simulink model "VirtualDAQ"  (R2021b)
settings: Solver=VariableStepAuto  StartTime=0.0  StopTime=inf  MaxStep=0.001  RelTol=1e-3
PostLoadFcn:
  | % Resize the model window
  | set(0,"Units","pixels")
  | sSize = get(0,"screensize");
  | set_param(gcs,'location',...
  |     [1,sSize(4)*0.01,round(sSize(3)/2),sSize(4)*0.96]);
  | 
  | % Reset the zoom
  | set_param(gcs, 'ZoomFactor','FitSystem')
libraries: fl_lib x5, simulink x4, nesl_utility x3, ee_lib x1, dspxfrm3 x1
(part 2 of 2)

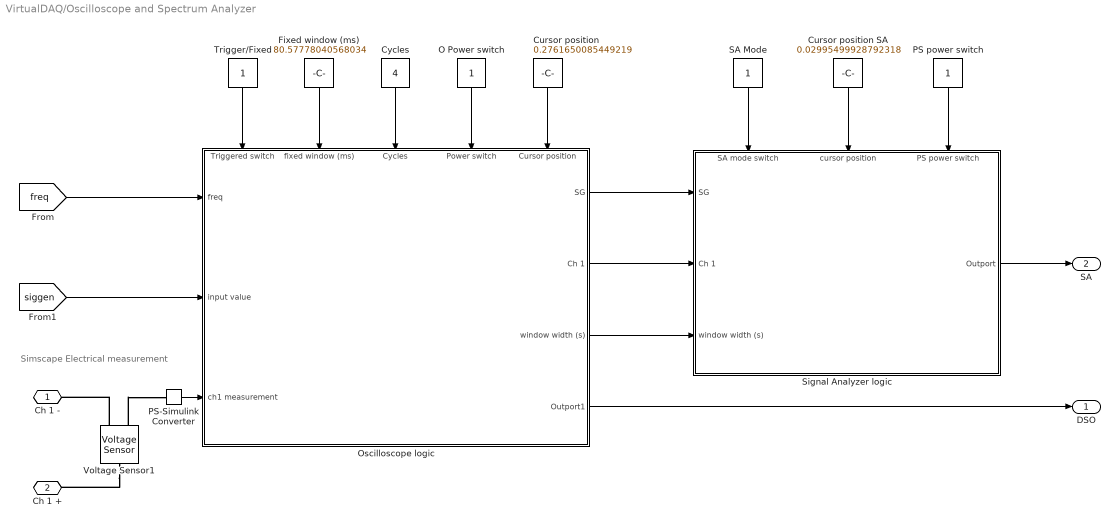
== system VirtualDAQ/Oscilloscope and Spectrum Analyzer ==
  note: Simscape Electrical
      | measurement
  Cursor position : Constant  Value=0.2761650085449219
  Cursor position SA : Constant  Value=0.02995499928792318
  Cycles : Constant  Value=4
  Fixed window (ms) : Constant  Value=80.57778040568034
  O Power switch : Constant
  Oscilloscope logic : Subsystem
      settings: PortSchema="{\"entries\":[{\"content\":{\"sides\":[{\"content\":{\"connectorIds\":[\"In1\",\"In2\",\"In3\"]},\"type\":\"ConnectorPlacement.EquallySpacedRectSide\",\"uuid\":\"f2d86859-c2b3-4aba-b253-ab7209c6bd09\"},{\"content\":{\"connectorIds\":[\"Out1\",\"Out2\",\"Out3\",\"Out4\"],\"side\":\"RIGHT\"},\"type\":\"ConnectorPlacement.EquallySpacedRectSide\",\"uuid\":\"576f7b6f-22d6-428c-bce1-54cbe46983a0\"},{\"content\":{\"connectorIds\":[\"In4\",\"In5\",\"In6\",\"In7\",\"In8\"],\"side\":\"TOP\"},\"type\":\"ConnectorPlacement.EquallySpacedRectSide\",\"uuid\":\"f25f0492-4e1a-4a19-8d4a-d023df9c7402\"}]},\"type\":\"ConnectorPlacement.EquallySpacedConnector\",\"uuid\":\"c0b076e3-46c8-476d-a521-4d4d737350f7\"}],\"packageUris\":[\"http://schema.mathworks.com/mf0/Connector/R2020b\"],\"version\":\"1.0\"}"
  PS power switch : Constant
  PS-Simulink Converter : nesl_utility/PS-Simulink Converter  PhysicalDomain=network_engine_domain  SubClassName=ps_output  LeftPortType=input  RightPortType=output  PseudoPeriodic=off  Frequencies=[]  Unit=inherit  AffineConversion=off
      settings: SourceProductBaseCode=PW,SS
  SA Mode : Constant
  Signal Analyzer logic : Subsystem
      settings: PortSchema="{\"entries\":[{\"content\":{\"sides\":[{\"content\":{\"connectorIds\":[\"In1\",\"In2\",\"In3\"]},\"type\":\"ConnectorPlacement.EquallySpacedRectSide\",\"uuid\":\"bb84044c-62d4-45e3-980b-d84da8bc32f8\"},{\"content\":{\"connectorIds\":[\"Out1\"],\"side\":\"RIGHT\"},\"type\":\"ConnectorPlacement.EquallySpacedRectSide\",\"uuid\":\"01e33b7c-25bd-4396-88e8-c83dc9c90d0e\"},{\"content\":{\"connectorIds\":[\"In4\",\"In5\",\"In6\"],\"side\":\"TOP\"},\"type\":\"ConnectorPlacement.EquallySpacedRectSide\",\"uuid\":\"0960ff1c-97c3-4c41-84a3-75686bdd4271\"}]},\"type\":\"ConnectorPlacement.EquallySpacedConnector\",\"uuid\":\"e23a09fd-d0ca-448f-9719-1e9fc283f1c0\"}],\"packageUris\":[\"http://schema.mathworks.com/mf0/Connector/R2020b\"],\"version\":\"1.0\"}"
  Trigger/Fixed : Constant
  Voltage Sensor1 : fl_lib/Electrical/Electrical Sensors/Voltage Sensor
  Ch 1 - : PMIOPort  Side=Left
  Ch 1 + : PMIOPort  Port=2  Side=Left
  DSO : Outport
  SA : Outport  Port=2
  wires:
  Trigger/Fixed/1 -> Oscilloscope logic/4(Triggered switch)
  Fixed window (ms)/1 -> Oscilloscope logic/5(fixed window (ms))
  Cycles/1 -> Oscilloscope logic/6(Cycles)
  O Power switch/1 -> Oscilloscope logic/7(Power switch)
  Cursor position/1 -> Oscilloscope logic/8(Cursor position)
  [freq] -> Oscilloscope logic/1(freq)
  [siggen] -> Oscilloscope logic/2(input value)
  Oscilloscope logic/4(Outport1) -> DSO/1
  SA Mode/1 -> Signal Analyzer logic/4(SA mode switch)
  Cursor position SA/1 -> Signal Analyzer logic/5(cursor position)
  PS power switch/1 -> Signal Analyzer logic/6(PS power switch)
  Oscilloscope logic/2(Ch 1) -> Signal Analyzer logic/2(Ch 1)
  Oscilloscope logic/1(SG) -> Signal Analyzer logic/1(SG)
  Oscilloscope logic/3(window width (s)) -> Signal Analyzer logic/3(window width (s))
  Signal Analyzer logic/1(Outport) -> SA/1
  PS-Simulink Converter/1 -> Oscilloscope logic/3(ch1 measurement)
  connections:
  Voltage Sensor1/RConn1 -- PS-Simulink Converter/LConn1
  Voltage Sensor1/LConn1 -- Ch 1 +/RConn1
  Voltage Sensor1/RConn2 -- Ch 1 -/RConn1

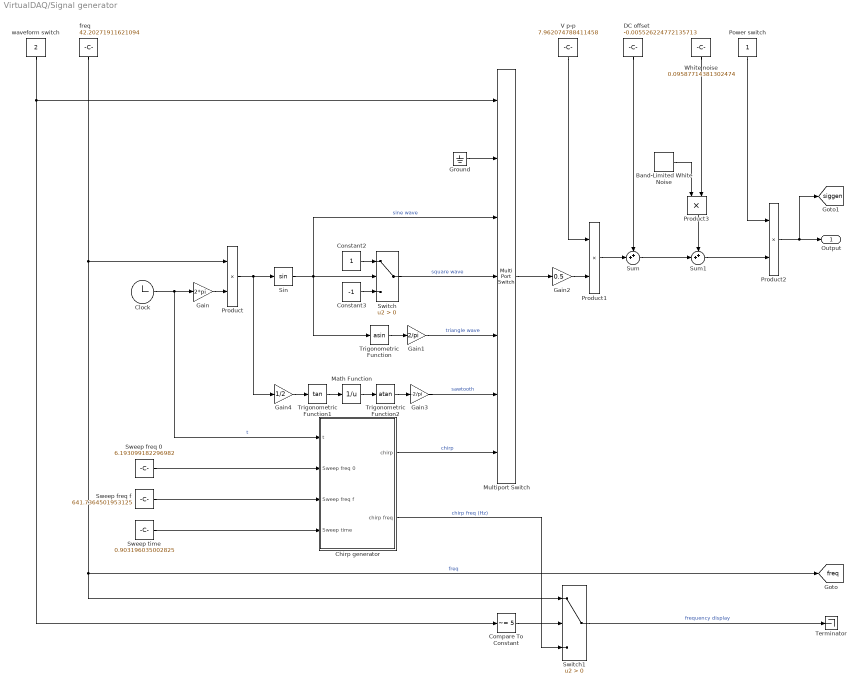
== system VirtualDAQ/Signal generator ==
  Band-Limited White Noise : simulink/Sources/Band-Limited White Noise  Cov=0.75e-6  Ts=0.5e-5  seed=[23341]
  Chirp generator : Subsystem
  Clock : Clock
  Compare To Constant : simulink/Logic and Bit Operations/Compare To Constant  relop=~=  const=5  OutDataTypeStr=boolean
  Constant2 : Constant  SampleTime=0
  Constant3 : Constant  Value=-1  SampleTime=0
  DC offset : Constant  Value=-0.005526224772135713
  Gain : Gain  Gain=2*pi
  Gain1 : Gain  Gain=2/pi
  Gain2 : Gain  Gain=0.5
  Gain3 : Gain  Gain=-2/pi
  Gain4 : Gain  Gain=1/2
  Ground : Ground
  Math Function : Math  Operator=reciprocal  SaturateOnIntegerOverflow=on
  Multiport Switch : MultiPortSwitch  DataPortOrder=Zero-based contiguous  Inputs=6  DiagnosticForDefault=None  zeroidx=on
  Power switch : Constant
  Product{,1..3} (4 alike) : Product
  Sin : Trigonometry
  Sum : Sum  Inputs=++|
  Sum1 : Sum  Inputs=++|
  Sweep freq 0 : Constant  Value=6.193099182296982
  Sweep freq f : Constant  Value=641.7364501953125
  Sweep time : Constant  Value=0.903196035002825
  Switch : Switch  Criteria=u2 > Threshold
  Switch1 : Switch  Criteria=u2 > Threshold
  Terminator : Terminator
  Trigonometric Function : Trigonometry  Operator=asin
  Trigonometric Function1 : Trigonometry  Operator=tan
  Trigonometric Function2 : Trigonometry  Operator=atan
  V p-p : Constant  Value=7.962074788411458  SampleTime=-1
  White noise : Constant  Value=0.09587714381302474
  freq : Constant  Value=42.20271911621094  SampleTime=0
  waveform switch : Constant  Value=2  SampleTime=0
  Output : Outport
  tag scope: freq=global, siggen=global
  wires:
  Sin/1 -> Multiport Switch/3, Trigonometric Function/1, Switch/2  "sine wave"
  freq/1 -> [freq], Switch1/1, Product/1  "freq"
  Clock/1 -> Chirp generator/1(t), Gain/1  "t"
  Ground/1 -> Multiport Switch/2
  Trigonometric Function/1 -> Gain1/1
  Constant2/1 -> Switch/1
  Constant3/1 -> Switch/3
  Gain2/1 -> Product1/2
  Product/1 -> Sin/1, Gain4/1
  Gain1/1 -> Multiport Switch/5  "triangle wave"
  Math Function/1 -> Trigonometric Function2/1
  Trigonometric Function1/1 -> Math Function/1
  Trigonometric Function2/1 -> Gain3/1
  Gain4/1 -> Trigonometric Function1/1
  Gain3/1 -> Multiport Switch/6  "sawtooth"
  V p-p/1 -> Product1/1
  Product1/1 -> Sum/2
  DC offset/1 -> Sum/1
  Switch/1 -> Multiport Switch/4  "square wave"
  Sum/1 -> Sum1/2
  Gain/1 -> Product/2
  Sweep time/1 -> Chirp generator/4(Sweep time)
  Chirp generator/1(chirp) -> Multiport Switch/7  "chirp"
  Sweep freq 0/1 -> Chirp generator/2(Sweep freq 0)
  Sweep freq f/1 -> Chirp generator/3(Sweep freq f)
  Compare To Constant/1 -> Switch1/2
  waveform switch/1 -> Compare To Constant/1, Multiport Switch/1
  Chirp generator/2(chirp freq) -> Switch1/3  "chirp freq (Hz)"
  Switch1/1 -> Terminator/1  "frequency display"
  Band-Limited White Noise/1 -> Product3/1
  White noise/1 -> Product3/2
  Product3/1 -> Sum1/1
  Power switch/1 -> Product2/1
  Sum1/1 -> Product2/2
  Product2/1 -> [siggen], Output/1
  Multiport Switch/1 -> Gain2/1

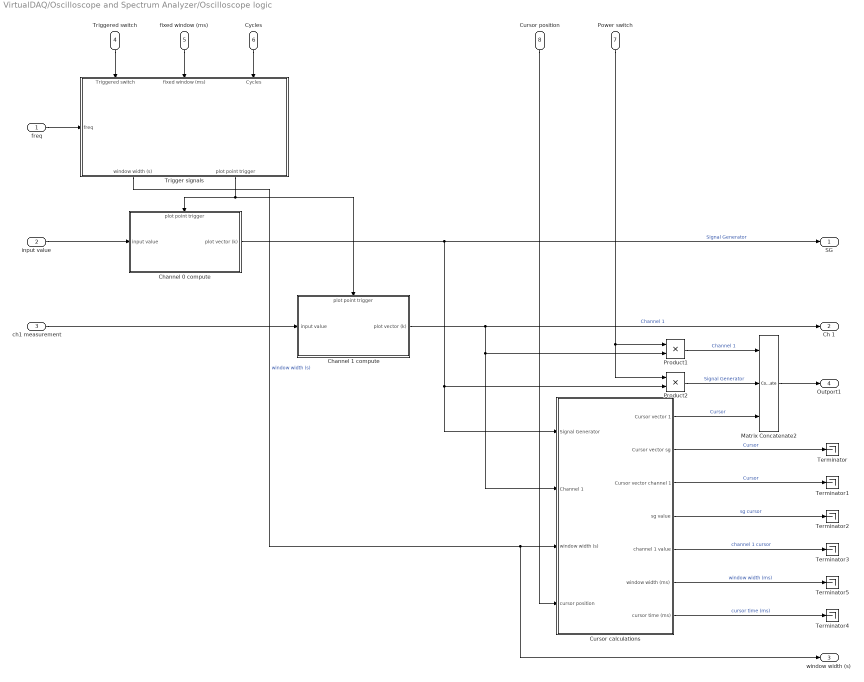
== system VirtualDAQ/Oscilloscope and Spectrum Analyzer/Oscilloscope logic ==
  freq : Inport
  input value : Inport  Port=2
  ch1 measurement : Inport  Port=3
  Triggered switch : Inport  Port=4
  fixed window (ms) : Inport  Port=5
  Cycles : Inport  Port=6
  Power switch : Inport  Port=7
  Cursor position : Inport  Port=8
  Channel 0 compute : Subsystem
      settings: PortSchema="{\"entries\":[{\"content\":{\"sides\":[{\"content\":{\"connectorIds\":[\"In1\"]},\"type\":\"ConnectorPlacement.EquallySpacedRectSide\",\"uuid\":\"56eea059-d5e9-4d95-b7d9-83a317b3103e\"},{\"content\":{\"connectorIds\":[\"Out1\"],\"side\":\"RIGHT\"},\"type\":\"ConnectorPlacement.EquallySpacedRectSide\",\"uuid\":\"fd8b8cd5-6def-4d8f-87ca-646372cc7fbe\"},{\"content\":{\"connectorIds\":[\"In2\"],\"side\":\"TOP\"},\"type\":\"ConnectorPlacement.EquallySpacedRectSide\",\"uuid\":\"3d9c38ee-b24b-466c-a7ac-a6d8a7456d51\"},{\"content\":{\"connectorIds\":[],\"side\":\"BOTTOM\"},\"type\":\"ConnectorPlacement.EquallySpacedRectSide\",\"uuid\":\"336136fa-2514-49ab-9e17-88caaca7366c\"}]},\"type\":\"ConnectorPlacement.EquallySpacedConnector\",\"uuid\":\"1d9824a8-6efd-49ff-b082-cf2ede19b4fd\"}],\"packageUris\":[\"http://schema.mathworks.com/mf0/Connector/R2020b\"],\"version\":\"1.0\"}"
  Channel 1 compute : Subsystem
      settings: PortSchema="{\"entries\":[{\"content\":{\"sides\":[{\"content\":{\"connectorIds\":[\"In1\"]},\"type\":\"ConnectorPlacement.EquallySpacedRectSide\",\"uuid\":\"56eea059-d5e9-4d95-b7d9-83a317b3103e\"},{\"content\":{\"connectorIds\":[\"Out1\"],\"side\":\"RIGHT\"},\"type\":\"ConnectorPlacement.EquallySpacedRectSide\",\"uuid\":\"fd8b8cd5-6def-4d8f-87ca-646372cc7fbe\"},{\"content\":{\"connectorIds\":[\"In2\"],\"side\":\"TOP\"},\"type\":\"ConnectorPlacement.EquallySpacedRectSide\",\"uuid\":\"3d9c38ee-b24b-466c-a7ac-a6d8a7456d51\"},{\"content\":{\"connectorIds\":[],\"side\":\"BOTTOM\"},\"type\":\"ConnectorPlacement.EquallySpacedRectSide\",\"uuid\":\"336136fa-2514-49ab-9e17-88caaca7366c\"}]},\"type\":\"ConnectorPlacement.EquallySpacedConnector\",\"uuid\":\"1d9824a8-6efd-49ff-b082-cf2ede19b4fd\"}],\"packageUris\":[\"http://schema.mathworks.com/mf0/Connector/R2020b\"],\"version\":\"1.0\"}"
  Cursor calculations : Subsystem
  Matrix Concatenate2 : Concatenate  NumInputs=3  Mode=Multidimensional array  ConcatenateDimension=2
  Product1 : Product
  Product2 : Product
  Terminator{,1..5} (6 alike) : Terminator
  Trigger signals : Subsystem
      settings: PortSchema="{\"entries\":[{\"content\":{\"sides\":[{\"content\":{\"connectorIds\":[\"In1\"]},\"type\":\"ConnectorPlacement.EquallySpacedRectSide\",\"uuid\":\"b92255b7-066e-487b-9e0c-e19692fc940f\"},{\"content\":{\"connectorIds\":[],\"side\":\"RIGHT\"},\"type\":\"ConnectorPlacement.EquallySpacedRectSide\",\"uuid\":\"cb964d42-f40b-466c-b45b-853437324272\"},{\"content\":{\"connectorIds\":[\"In2\",\"In3\",\"In4\"],\"side\":\"TOP\"},\"type\":\"ConnectorPlacement.EquallySpacedRectSide\",\"uuid\":\"e1027385-b295-47a3-ae7d-2e3bb07fa1de\"},{\"content\":{\"connectorIds\":[\"Out1\",\"Out2\"],\"side\":\"BOTTOM\"},\"type\":\"ConnectorPlacement.EquallySpacedRectSide\",\"uuid\":\"c27dc584-c0ba-4e72-b8bf-7374d1985911\"}]},\"type\":\"ConnectorPlacement.EquallySpacedConnector\",\"uuid\":\"1db11e79-2cf0-4841-86d9-651820ebc8ee\"}],\"packageUris\":[\"http://schema.mathworks.com/mf0/Connector/R2020b\"],\"version\":\"1.0\"}"
  SG : Outport
  Ch 1 : Outport  Port=2
  window width (s) : Outport  Port=3
  Outport1 : Outport  Port=4
  wires:
  Channel 0 compute/1(plot vector (k)) -> Cursor calculations/1(Signal Generator), Product2/2, SG/1  "Signal Generator"
  Power switch/1 -> Product2/1, Product1/1
  Trigger signals/2(plot point trigger) -> Channel 0 compute/2(plot point trigger), Channel 1 compute/2(plot point trigger)
  Trigger signals/1(window width (s)) -> window width (s)/1, Cursor calculations/3(window width (s))  "window width (s)"
  Channel 1 compute/1(plot vector (k)) -> Cursor calculations/2(Channel 1), Product1/2, Ch 1/1  "Channel 1"
  Cursor calculations/2(Cursor vector sg) -> Terminator/1  "Cursor"
  Cursor calculations/7(cursor time (ms)) -> Terminator4/1  "cursor time (ms)"
  Cursor calculations/4(sg value) -> Terminator2/1  "sg cursor"
  Cursor calculations/3(Cursor vector channel 1) -> Terminator1/1  "Cursor"
  Cursor calculations/5(channel 1 value) -> Terminator3/1  "channel 1 cursor"
  fixed window (ms)/1 -> Trigger signals/3(fixed window (ms))
  Cursor calculations/1(Cursor vector 1) -> Matrix Concatenate2/3  "Cursor"
  Product1/1 -> Matrix Concatenate2/1  "Channel 1"
  Cursor calculations/6(window width (ms)) -> Terminator5/1  "window width (ms)"
  Product2/1 -> Matrix Concatenate2/2  "Signal Generator"
  Triggered switch/1 -> Trigger signals/2(Triggered switch)
  input value/1 -> Channel 0 compute/1(input value)
  Cycles/1 -> Trigger signals/4(Cycles)
  freq/1 -> Trigger signals/1(freq)
  Matrix Concatenate2/1 -> Outport1/1
  Cursor position/1 -> Cursor calculations/4(cursor position)
  ch1 measurement/1 -> Channel 1 compute/1(input value)

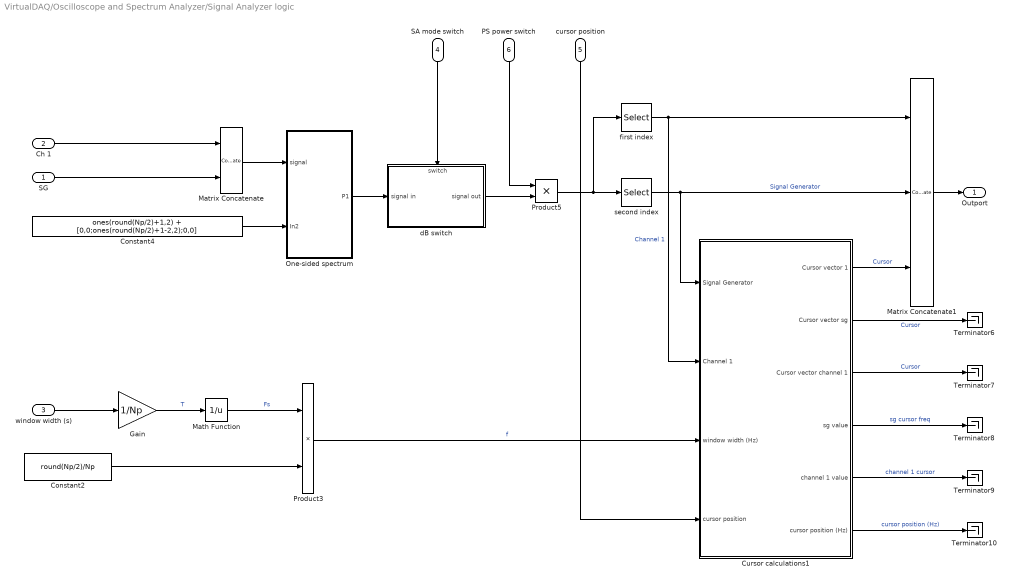
== system VirtualDAQ/Oscilloscope and Spectrum Analyzer/Signal Analyzer logic ==
  SG : Inport
  Ch 1 : Inport  Port=2
  window width (s) : Inport  Port=3
  SA mode switch : Inport  Port=4
  cursor position : Inport  Port=5
  PS power switch : Inport  Port=6
  Constant2 : Constant  Value=round(Np/2)/Np
  Constant4 : Constant  Value=ones(round(Np/2)+1,2) + [0,0;ones(round(Np/2)+1-2,2);0,0]
  Cursor calculations1 : Subsystem
  Gain : Gain  Gain=1/Np
  Math Function : Math  Operator=reciprocal  SaturateOnIntegerOverflow=on
  Matrix Concatenate : Concatenate  Mode=Multidimensional array  ConcatenateDimension=2
  Matrix Concatenate1 : Concatenate  NumInputs=3  Mode=Multidimensional array  ConcatenateDimension=2
  One-sided spectrum : Subsystem
  Product3 : Product
  Product5 : Product
  Terminator{6..10} (5 alike) : Terminator
  dB switch : Subsystem
      settings: PortSchema="{\"entries\":[{\"content\":{\"sides\":[{\"content\":{\"connectorIds\":[\"In1\"]},\"type\":\"ConnectorPlacement.EquallySpacedRectSide\",\"uuid\":\"731d6ea0-13ec-4437-83d3-031943873cb5\"},{\"content\":{\"connectorIds\":[\"Out1\"],\"side\":\"RIGHT\"},\"type\":\"ConnectorPlacement.EquallySpacedRectSide\",\"uuid\":\"4a6928d1-e59a-43a6-b645-c5c732165a4d\"},{\"content\":{\"connectorIds\":[\"In2\"],\"side\":\"TOP\"},\"type\":\"ConnectorPlacement.EquallySpacedRectSide\",\"uuid\":\"01c58549-3c91-47fa-983a-e1347000b7e8\"}]},\"type\":\"ConnectorPlacement.EquallySpacedConnector\",\"uuid\":\"72ae96ee-473e-47d4-a3f7-467fafe8904d\"}],\"packageUris\":[\"http://schema.mathworks.com/mf0/Connector/R2020b\"],\"version\":\"1.0\"}"
  first index : Selector  NumberOfDimensions=2  InputPortWidth=3  IndexOptions=Select all,Index vector (dialog)  Indices=[1 3],1  OutputSizes=1,1
  second index : Selector  NumberOfDimensions=2  InputPortWidth=3  IndexOptions=Select all,Index vector (dialog)  Indices=[1 3],2  OutputSizes=1,1
  Outport : Outport
  wires:
  Constant2/1 -> Product3/2
  Math Function/1 -> Product3/1  "Fs"
  Gain/1 -> Math Function/1  "T"
  Product3/1 -> Cursor calculations1/3(window width (Hz))  "f"
  Cursor calculations1/6(cursor position (Hz)) -> Terminator10/1  "cursor position (Hz)"
  Matrix Concatenate/1 -> One-sided spectrum/1(signal)
  first index/1 -> Cursor calculations1/2(Channel 1), Matrix Concatenate1/1  "Channel 1"
  Cursor calculations1/5(channel 1 value) -> Terminator9/1  "channel 1 cursor"
  Cursor calculations1/1(Cursor vector 1) -> Matrix Concatenate1/3  "Cursor"
  second index/1 -> Matrix Concatenate1/2, Cursor calculations1/1(Signal Generator)  "Signal Generator"
  Constant4/1 -> One-sided spectrum/2(In2)
  Cursor calculations1/3(Cursor vector channel 1) -> Terminator7/1  "Cursor"
  window width (s)/1 -> Gain/1
  Product5/1 -> first index/1, second index/1
  PS power switch/1 -> Product5/1
  One-sided spectrum/1(P1) -> dB switch/1(signal in)
  Cursor calculations1/4(sg value) -> Terminator8/1  "sg cursor freq"
  Cursor calculations1/2(Cursor vector sg) -> Terminator6/1  "Cursor"
  SG/1 -> Matrix Concatenate/2
  dB switch/1(signal out) -> Product5/2
  Ch 1/1 -> Matrix Concatenate/1
  cursor position/1 -> Cursor calculations1/4(cursor position)
  SA mode switch/1 -> dB switch/2(switch)
  Matrix Concatenate1/1 -> Outport/1

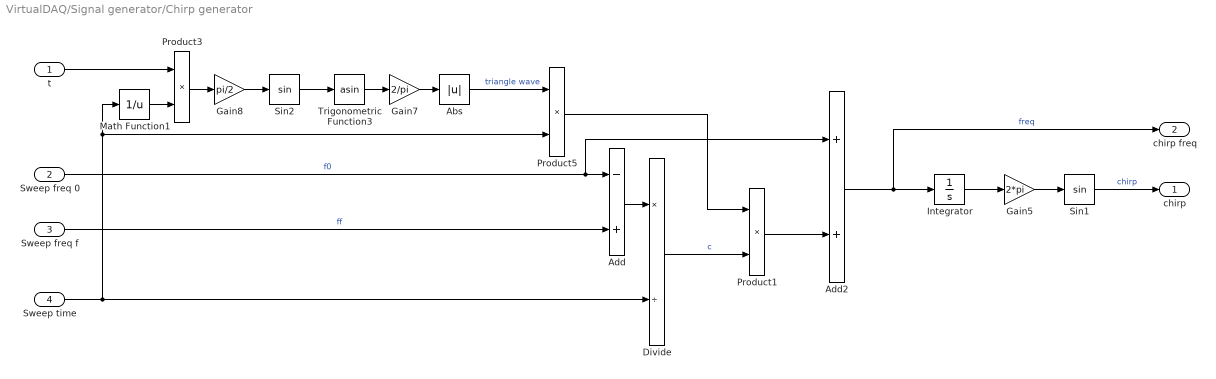
== system VirtualDAQ/Signal generator/Chirp generator ==
  t : Inport
  Sweep freq 0 : Inport  Port=2
  Sweep freq f : Inport  Port=3
  Sweep time : Inport  Port=4
  Abs : Abs
  Add : Sum  Inputs=-+
  Add2 : Sum
  Divide : Product  Inputs=*/
  Gain5 : Gain  Gain=2*pi
  Gain7 : Gain  Gain=2/pi
  Gain8 : Gain  Gain=pi/2
  Integrator : Integrator
  Math Function1 : Math  Operator=reciprocal  SaturateOnIntegerOverflow=on
  Product1 : Product
  Product3 : Product
  Product5 : Product
  Sin1 : Trigonometry
  Sin2 : Trigonometry
  Trigonometric Function3 : Trigonometry  Operator=asin
  chirp : Outport
  chirp freq : Outport  Port=2
  wires:
  Add/1 -> Divide/1
  Gain5/1 -> Sin1/1
  Gain8/1 -> Sin2/1
  Divide/1 -> Product1/2  "c"
  Sweep time/1 -> Divide/2, Product5/2, Math Function1/1
  Gain7/1 -> Abs/1
  t/1 -> Product3/1
  Sin2/1 -> Trigonometric Function3/1
  Trigonometric Function3/1 -> Gain7/1
  Math Function1/1 -> Product3/2
  Sin1/1 -> chirp/1  "chirp"
  Sweep freq 0/1 -> Add2/1, Add/1  "f0"
  Sweep freq f/1 -> Add/2  "ff"
  Product1/1 -> Add2/2
  Integrator/1 -> Gain5/1
  Add2/1 -> chirp freq/1, Integrator/1  "freq"
  Product3/1 -> Gain8/1
  Abs/1 -> Product5/1  "triangle wave"
  Product5/1 -> Product1/1

== system VirtualDAQ/Oscilloscope and Spectrum Analyzer/Oscilloscope logic/Channel 0 compute ==
  note: This level stores the plot values inside the delay block
  input value : Inport
  plot point trigger : Inport  Port=2
  Rate Transition2 : RateTransition  InitialCondition=zeros(Np,1)  OutPortSampleTime=1/refreshRate
  Triggered Subsystem : Subsystem  TreatAsAtomicUnit=on
  plot vector values : UnitDelay  InitialCondition=zeros(Np,1)  SampleTime=-1  HasFrameUpgradeWarning=on
  plot vector (k) : Outport
  wires:
  plot point trigger/1 -> Triggered Subsystem/Trigger
  Triggered Subsystem/1(plot vector (k)) -> Rate Transition2/1, plot vector values/1
  input value/1 -> Triggered Subsystem/1(input value)
  Rate Transition2/1 -> plot vector (k)/1
  plot vector values/1 -> Triggered Subsystem/2(plot vector (k-1))

== system VirtualDAQ/Oscilloscope and Spectrum Analyzer/Oscilloscope logic/Channel 1 compute ==
  note: This level stores the plot values inside the delay block
  input value : Inport
  plot point trigger : Inport  Port=2
  Rate Transition2 : RateTransition  InitialCondition=zeros(Np,1)  OutPortSampleTime=1/refreshRate
  Triggered Subsystem : Subsystem  TreatAsAtomicUnit=on
  plot vector values : UnitDelay  InitialCondition=zeros(Np,1)  SampleTime=-1  HasFrameUpgradeWarning=on
  plot vector (k) : Outport
  wires:
  plot point trigger/1 -> Triggered Subsystem/Trigger
  Triggered Subsystem/1(plot vector (k)) -> Rate Transition2/1, plot vector values/1
  input value/1 -> Triggered Subsystem/1(input value)
  Rate Transition2/1 -> plot vector (k)/1
  plot vector values/1 -> Triggered Subsystem/2(plot vector (k-1))

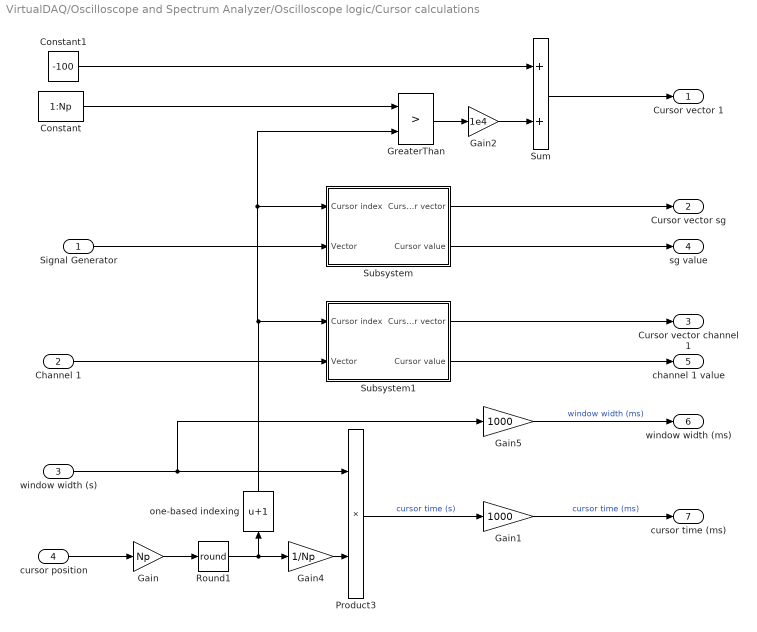
== system VirtualDAQ/Oscilloscope and Spectrum Analyzer/Oscilloscope logic/Cursor calculations ==
  Signal Generator : Inport
  Channel 1 : Inport  Port=2
  window width (s) : Inport  Port=3
  cursor position : Inport  Port=4
  Constant : Constant  Value=1:Np
  Constant1 : Constant  Value=-100
  Gain : Gain  Gain=Np
  Gain1 : Gain  Gain=1000
  Gain2 : Gain  Gain=1e4
  Gain4 : Gain  Gain=1/Np
  Gain5 : Gain  Gain=1000
  GreaterThan : RelationalOperator  Operator=>  OutDataTypeStr=boolean  RndMeth=Simplest
  Product3 : Product
  Round1 : Rounding  Operator=round
  Subsystem : Subsystem
  Subsystem1 : Subsystem
  Sum : Sum
  one-based indexing : Bias  Bias=1
  Cursor vector 1 : Outport
  Cursor vector sg : Outport  Port=2
  Cursor vector channel 1 : Outport  Port=3
  sg value : Outport  Port=4
  channel 1 value : Outport  Port=5
  window width (ms) : Outport  Port=6
  cursor time (ms) : Outport  Port=7
  wires:
  cursor position/1 -> Gain/1
  Constant/1 -> GreaterThan/1
  Product3/1 -> Gain1/1  "cursor time (s)"
  Gain1/1 -> cursor time (ms)/1  "cursor time (ms)"
  GreaterThan/1 -> Gain2/1
  Sum/1 -> Cursor vector 1/1
  Gain2/1 -> Sum/2
  Subsystem1/2(Cursor value) -> channel 1 value/1
  Constant1/1 -> Sum/1
  Gain/1 -> Round1/1
  Gain4/1 -> Product3/2
  Channel 1/1 -> Subsystem1/2(Vector)
  Subsystem1/1("Cursor vector ") -> Cursor vector channel 1/1
  Round1/1 -> Gain4/1, one-based indexing/1
  window width (s)/1 -> Gain5/1, Product3/1
  Gain5/1 -> window width (ms)/1  "window width (ms)"
  Signal Generator/1 -> Subsystem/2(Vector)
  Subsystem/1("Cursor vector ") -> Cursor vector sg/1
  Subsystem/2(Cursor value) -> sg value/1
  one-based indexing/1 -> GreaterThan/2, Subsystem/1(Cursor index), Subsystem1/1(Cursor index)

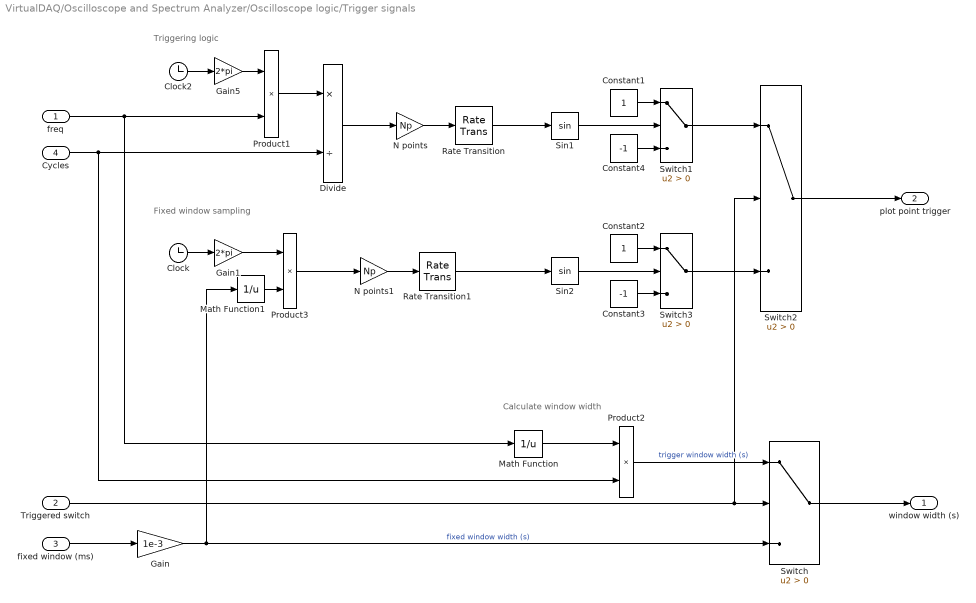
== system VirtualDAQ/Oscilloscope and Spectrum Analyzer/Oscilloscope logic/Trigger signals ==
  note: Calculate window width
  note: Triggering logic
  note: Fixed window sampling
  freq : Inport
  Triggered switch : Inport  Port=2
  fixed window (ms) : Inport  Port=3
  Cycles : Inport  Port=4
  Clock : Clock
  Clock2 : Clock
  Constant1 : Constant  SampleTime=0
  Constant2 : Constant  SampleTime=0
  Constant3 : Constant  Value=-1  SampleTime=0
  Constant4 : Constant  Value=-1  SampleTime=0
  Divide : Product  Inputs=*/
  Gain : Gain  Gain=1e-3
  Gain1 : Gain  Gain=2*pi
  Gain5 : Gain  Gain=2*pi
  Math Function : Math  Operator=reciprocal  SaturateOnIntegerOverflow=on
  Math Function1 : Math  Operator=reciprocal  SaturateOnIntegerOverflow=on
  N points : Gain  Gain=Np
  N points1 : Gain  Gain=Np
  Product1 : Product
  Product2 : Product
  Product3 : Product
  Rate Transition : RateTransition  OutPortSampleTime=plot_dt
  Rate Transition1 : RateTransition  OutPortSampleTime=plot_dt
  Sin1 : Trigonometry
  Sin2 : Trigonometry
  Switch{,1..3} (4 alike) : Switch  Criteria=u2 > Threshold
  window width (s) : Outport
  plot point trigger : Outport  Port=2
  wires:
  Gain5/1 -> Product1/1
  Constant4/1 -> Switch1/3
  Clock2/1 -> Gain5/1
  Sin1/1 -> Switch1/2
  Constant1/1 -> Switch1/1
  Product1/1 -> Divide/1
  Divide/1 -> N points/1
  N points/1 -> Rate Transition/1
  Rate Transition/1 -> Sin1/1
  Switch2/1 -> plot point trigger/1
  Triggered switch/1 -> Switch/2, Switch2/2
  Product2/1 -> Switch/1  "trigger window width (s)"
  freq/1 -> Product1/2, Math Function/1
  Cycles/1 -> Divide/2, Product2/2
  Math Function/1 -> Product2/1
  fixed window (ms)/1 -> Gain/1
  Switch/1 -> window width (s)/1
  Switch1/1 -> Switch2/1
  N points1/1 -> Rate Transition1/1
  Constant2/1 -> Switch3/1
  Sin2/1 -> Switch3/2
  Constant3/1 -> Switch3/3
  Switch3/1 -> Switch2/3
  Rate Transition1/1 -> Sin2/1
  Clock/1 -> Gain1/1
  Product3/1 -> N points1/1
  Gain/1 -> Math Function1/1, Switch/3  "fixed window width (s)"
  Gain1/1 -> Product3/1
  Math Function1/1 -> Product3/2

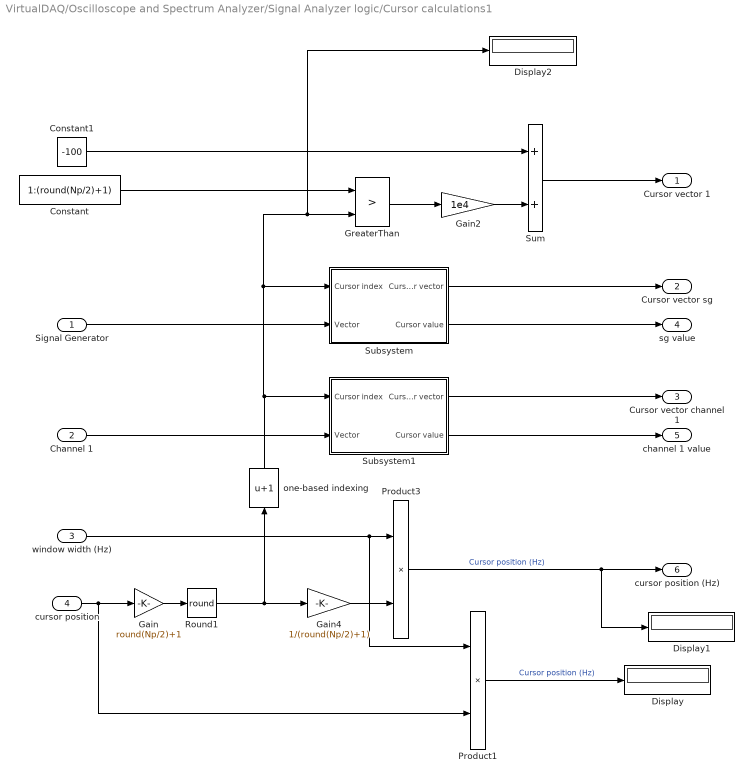
== system VirtualDAQ/Oscilloscope and Spectrum Analyzer/Signal Analyzer logic/Cursor calculations1 ==
  Signal Generator : Inport
  Channel 1 : Inport  Port=2
  window width (Hz) : Inport  Port=3
  cursor position : Inport  Port=4
  Constant : Constant  Value=1:(round(Np/2)+1)
  Constant1 : Constant  Value=-100
  Display : Display
  Display1 : Display
  Display2 : Display
  Gain : Gain  Gain=round(Np/2)+1
  Gain2 : Gain  Gain=1e4
  Gain4 : Gain  Gain=1/(round(Np/2)+1)
  GreaterThan : RelationalOperator  Operator=>  OutDataTypeStr=boolean  RndMeth=Simplest
  Product1 : Product
  Product3 : Product
  Round1 : Rounding  Operator=round
  Subsystem : Subsystem
  Subsystem1 : Subsystem
  Sum : Sum
  one-based indexing : Bias  Bias=1
  Cursor vector 1 : Outport
  Cursor vector sg : Outport  Port=2
  Cursor vector channel 1 : Outport  Port=3
  sg value : Outport  Port=4
  channel 1 value : Outport  Port=5
  cursor position (Hz) : Outport  Port=6
  wires:
  cursor position/1 -> Gain/1, Product1/2
  Constant/1 -> GreaterThan/1
  Product3/1 -> Display1/1, cursor position (Hz)/1  "Cursor position (Hz)"
  GreaterThan/1 -> Gain2/1
  Gain2/1 -> Sum/2
  Subsystem1/2(Cursor value) -> channel 1 value/1
  Constant1/1 -> Sum/1
  Gain/1 -> Round1/1
  Channel 1/1 -> Subsystem1/2(Vector)
  Subsystem1/1("Cursor vector ") -> Cursor vector channel 1/1
  Round1/1 -> Gain4/1, one-based indexing/1
  Signal Generator/1 -> Subsystem/2(Vector)
  Subsystem/1("Cursor vector ") -> Cursor vector sg/1
  Subsystem/2(Cursor value) -> sg value/1
  Sum/1 -> Cursor vector 1/1
  Gain4/1 -> Product3/2
  window width (Hz)/1 -> Product1/1, Product3/1
  Product1/1 -> Display/1  "Cursor position (Hz)"
  one-based indexing/1 -> Display2/1, GreaterThan/2, Subsystem/1(Cursor index), Subsystem1/1(Cursor index)

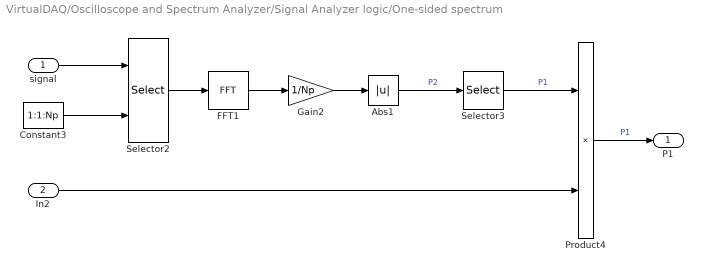
== system VirtualDAQ/Oscilloscope and Spectrum Analyzer/Signal Analyzer logic/One-sided spectrum ==
  signal : Inport
  In2 : Inport  Port=2
  Abs1 : Abs
  Constant3 : Constant  Value=1:1:Np
  FFT1 : dspxfrm3/FFT  FFTImplementation=Auto  CompMethod=Table lookup  TableOpt=NEW  TableOptActive=Speed  BitRevOrder=off  Normalize=off  InheritFFTLength=on  FFTLength=64  WrapInput=on  roundingMode=Floor  overflowMode=off  firstCoeffDataTypeStr=Inherit: Same word length as input  firstCoeffLastDataTypeStr=Inherit: Same word length as input  outputMin=[]  outputMax=[]
  Gain2 : Gain  Gain=1/Np
  Product4 : Product
  Selector2 : Selector  NumberOfDimensions=2  InputPortWidth=Np  IndexOptions=Index vector (port),Select all  Indices=1:4:Np,1  OutputSizes=1,1
  Selector3 : Selector  NumberOfDimensions=2  InputPortWidth=Np  IndexOptions=Index vector (dialog),Select all  Indices=1:round(Np/2)+1,1  OutputSizes=1,1
  P1 : Outport
  wires:
  Constant3/1 -> Selector2/2
  Selector2/1 -> FFT1/1
  FFT1/1 -> Gain2/1
  Gain2/1 -> Abs1/1
  In2/1 -> Product4/2
  Abs1/1 -> Selector3/1  "P2"
  signal/1 -> Selector2/1
  Selector3/1 -> Product4/1  "P1"
  Product4/1 -> P1/1  "P1"

== system VirtualDAQ/Oscilloscope and Spectrum Analyzer/Signal Analyzer logic/dB switch ==
  signal in : Inport
  switch : Inport  Port=2
  Gain3 : Gain  Gain=10
  Log2 : Math  Operator=log10  SaturateOnIntegerOverflow=on
  Switch2 : Switch  Criteria=u2 > Threshold
  signal out : Outport
  wires:
  Gain3/1 -> Switch2/3  "P1 in dB"
  Switch2/1 -> signal out/1
  Log2/1 -> Gain3/1
  signal in/1 -> Log2/1, Switch2/1
  switch/1 -> Switch2/2

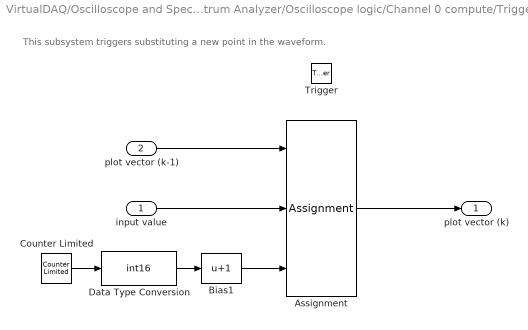
== system VirtualDAQ/Oscilloscope and Spectrum Analyzer/Oscilloscope logic/Channel 0 compute/Triggered Subsystem ==
  note: This subsystem triggers substituting a new point in the waveform.
  input value : Inport
  plot vector (k-1) : Inport  Port=2
  Trigger : TriggerPort  VariantControl=(inherit)
  Assignment : Assignment  DiagnosticForDimensions=Warning  IndexOptions=Index vector (port)  Indices=1  OutputSizes=1
  Bias1 : Bias  Bias=1
  Counter Limited : simulink/Sources/Counter Limited  uplimit=Np-1  tsamp=-1
  Data Type Conversion : DataTypeConversion  OutDataTypeStr=int16
  plot vector (k) : Outport
  wires:
  Assignment/1 -> plot vector (k)/1
  input value/1 -> Assignment/2
  Counter Limited/1 -> Data Type Conversion/1
  Bias1/1 -> Assignment/3
  plot vector (k-1)/1 -> Assignment/1
  Data Type Conversion/1 -> Bias1/1

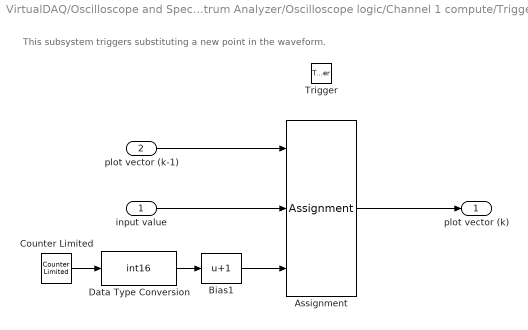
== system VirtualDAQ/Oscilloscope and Spectrum Analyzer/Oscilloscope logic/Channel 1 compute/Triggered Subsystem ==
  note: This subsystem triggers substituting a new point in the waveform.
  input value : Inport
  plot vector (k-1) : Inport  Port=2
  Trigger : TriggerPort  VariantControl=(inherit)
  Assignment : Assignment  DiagnosticForDimensions=Warning  IndexOptions=Index vector (port)  Indices=1  OutputSizes=1
  Bias1 : Bias  Bias=1
  Counter Limited : simulink/Sources/Counter Limited  uplimit=Np-1  tsamp=-1
  Data Type Conversion : DataTypeConversion  OutDataTypeStr=int16
  plot vector (k) : Outport
  wires:
  Assignment/1 -> plot vector (k)/1
  input value/1 -> Assignment/2
  Counter Limited/1 -> Data Type Conversion/1
  Bias1/1 -> Assignment/3
  plot vector (k-1)/1 -> Assignment/1
  Data Type Conversion/1 -> Bias1/1

== system VirtualDAQ/Oscilloscope and Spectrum Analyzer/Oscilloscope logic/Cursor calculations/Subsystem ==
  Cursor index : Inport
  Vector : Inport  Port=2
  Assignment1 : Assignment  DiagnosticForDimensions=Warning  IndexOptions=Index vector (port)  Indices=1  OutputSizes=1
  Constant2 : Constant  Value=nan(Np,1)
  Selector : Selector  InputPortWidth=Np  IndexOptions=Index vector (port)  Indices=[1 3]  OutputSizes=1
  "Cursor vector " : Outport
  Cursor value : Outport  Port=2
  wires:
  Selector/1 -> Cursor value/1, Assignment1/2
  Assignment1/1 -> "Cursor vector "/1
  Cursor index/1 -> Selector/2, Assignment1/3
  Vector/1 -> Selector/1
  Constant2/1 -> Assignment1/1

== system VirtualDAQ/Oscilloscope and Spectrum Analyzer/Oscilloscope logic/Cursor calculations/Subsystem1 ==
  Cursor index : Inport
  Vector : Inport  Port=2
  Assignment1 : Assignment  DiagnosticForDimensions=Warning  IndexOptions=Index vector (port)  Indices=1  OutputSizes=1
  Constant2 : Constant  Value=nan(Np,1)
  Selector : Selector  InputPortWidth=Np  IndexOptions=Index vector (port)  Indices=[1 3]  OutputSizes=1
  "Cursor vector " : Outport
  Cursor value : Outport  Port=2
  wires:
  Selector/1 -> Cursor value/1, Assignment1/2
  Assignment1/1 -> "Cursor vector "/1
  Cursor index/1 -> Selector/2, Assignment1/3
  Vector/1 -> Selector/1
  Constant2/1 -> Assignment1/1

== system VirtualDAQ/Oscilloscope and Spectrum Analyzer/Signal Analyzer logic/Cursor calculations1/Subsystem ==
  Cursor index : Inport
  Vector : Inport  Port=2
  Assignment1 : Assignment  DiagnosticForDimensions=Warning  IndexOptions=Index vector (port)  Indices=1  OutputSizes=1
  Constant2 : Constant  Value=nan(round(Np/2)+1,1)
  Selector : Selector  InputPortWidth=round(Np/2)+1  IndexOptions=Index vector (port)  Indices=[1 3]  OutputSizes=1
  "Cursor vector " : Outport
  Cursor value : Outport  Port=2
  wires:
  Selector/1 -> Cursor value/1, Assignment1/2
  Assignment1/1 -> "Cursor vector "/1
  Cursor index/1 -> Selector/2, Assignment1/3
  Vector/1 -> Selector/1
  Constant2/1 -> Assignment1/1

== system VirtualDAQ/Oscilloscope and Spectrum Analyzer/Signal Analyzer logic/Cursor calculations1/Subsystem1 ==
  Cursor index : Inport
  Vector : Inport  Port=2
  Assignment1 : Assignment  DiagnosticForDimensions=Warning  IndexOptions=Index vector (port)  Indices=1  OutputSizes=1
  Constant2 : Constant  Value=nan(round(Np/2)+1,1)
  Selector : Selector  InputPortWidth=round(Np/2)+1  IndexOptions=Index vector (port)  Indices=[1 3]  OutputSizes=1
  "Cursor vector " : Outport
  Cursor value : Outport  Port=2
  wires:
  Selector/1 -> Cursor value/1, Assignment1/2
  Assignment1/1 -> "Cursor vector "/1
  Cursor index/1 -> Selector/2, Assignment1/3
  Vector/1 -> Selector/1
  Constant2/1 -> Assignment1/1
